simulink model "gm_external_state_machine"  (R2021a)
settings: Solver=FixedStepDiscrete  StartTime=0.0  StopTime=200*t_ADC  RelTol=1e-3
undefined symbols (not defined in the file or in its folder): A, IB, id_ref, iq_ref, ix_ref, iy_ref, lambda_d, lambda_q, lambda_u, lambda_x, lambda_y, Ld_over_LB, Lq_over_LB, n_rpm, omega_m, omegaB, p, psi_pm_over_psiB, Rs_over_ZB, t_ADC, t_clock, Ts_times_ZB_over_Ld, Ts_times_ZB_over_Lq, Ts_times_ZB_over_Lx, Ts_times_ZB_over_Ly, v_dc, VB
libraries: nesl_utility x38, fl_lib x30, simulink x19, ee_lib x14, hdlsllib x4, spsAlphaBetaZerotodq0Lib x1
(part 1 of 4)
settings Model: Creator=micha  LastModifiedBy=micha
settings SolverCC: AlgebraicLoopSolver=TrustRegion
settings DataIOCC: LimitDataPoints=on  SaveOutput=off  SaveTime=off
settings OptimizationCC: BlockReduction=off  ConditionallyExecuteInputs=off  DefaultParameterBehavior=Inlined  LifeSpan=inf
settings DebuggingCC: AlgebraicLoopMsg=error  InheritedTsInSrcMsg=none  SingleTaskRateTransMsg=error  AllowSymbolicDim=off  StrictBusMsg=ErrorOnBusTreatedAsVector  SFUnexpectedBacktrackingDiag=warning  SFNoUnconditionalDefaultTransitionDiag=warning  SFExecutionAtInitializationDiag=none  SFMachineParentedDataDiag=warning  ArithmeticOperatorsInVariantConditions=warning
settings HardwareCC: ProdBitPerPointer=32  ProdBitPerSizeT=32  ProdBitPerPtrDiffT=32  ProdLargestAtomicFloat=None  ProdIntDivRoundTo=Undefined  ProdEndianess=Unspecified  ProdWordSize=32  ProdHWDeviceType=ASIC/FPGA->ASIC/FPGA  ProdEqTarget=off
settings SFSimCC: SimUseLocalCustomCode=off  CustomCodeUndefinedFunction=UseInterfaceOnly
settings RTWCC: RTWUseLocalCustomCode=off
settings CodeAppCC: StateflowObjectComments=on
settings GRTTargetCC: TargetLangStandard=C89/C90 (ANSI)
settings ConfigComp: CovScope=ReferencedModels  CovMetricSettings=dw  CovSaveCumulativeToWorkspaceVar=on  CovSaveSingleToWorkspaceVar=on  CovExternalEMLEnable=off  CovSFcnEnable=off

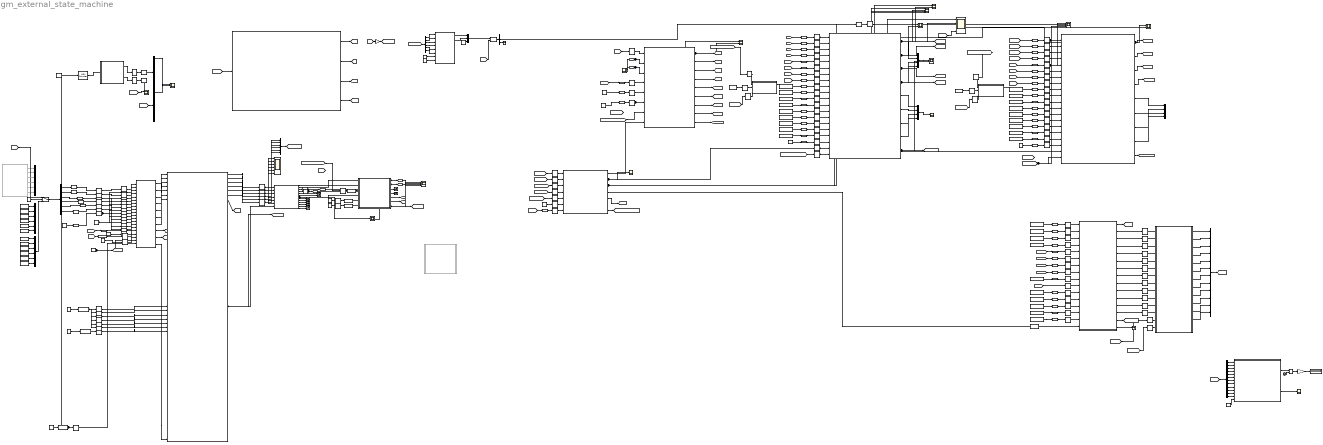
== system gm_external_state_machine ==
  note: 0=AXI 1=PL
  note: 1=sine source, 2=const
  note: check if timing is correct with delay done trigger
  note: 5 steps delay for xy currents, since dq transformation of alpha beta currents takes 5 clock steps. This way, the delay of dq is compensated
  6ph_PMSM_30deg_VSD1 : MATLAB Function  TreatAsAtomicUnit=on
  Alpha-Beta-Zero to dq1 : spsAlphaBetaZerotodq0Lib/Alpha-Beta-Zero to dq0  Alignment=Aligned with phase A axis
      settings: SourceProductBaseCode=PS
  Clock : Clock
  Constant : Constant  Value=64  OutDataTypeStr=uint32  SampleTime=-1
  Constant1 : Constant  Value=5
  Constant10 : Constant  Value=psi_pm_over_psiB
  Constant11 : Constant  Value=0.36
  Constant{12,45..50,52} (8 alike) : Constant  Value=0
  Constant13 : Constant  Value=5
  Constant14 : Constant  Value=psi_pm_over_psiB
  Constant15 : Constant  Value=Rs_over_ZB
  Constant16 : Constant  Value=omega_m/omegaB
  Constant17 : Constant  Value=Ts_times_ZB_over_Ld
  Constant18 : Constant  Value=Ts_times_ZB_over_Lq
  Constant19 : Constant  Value=Ts_times_ZB_over_Lx
  Constant{2,25,41,51} (4 alike) : Constant
  Constant20 : Constant  Value=Ts_times_ZB_over_Ly
  Constant21 : Constant  Value=Ld_over_LB
  Constant22 : Constant  Value=Lq_over_LB
  Constant23 : Constant  Value=omega_m/omegaB
  Constant24 : Constant  Value=1/3
  Constant26 : Constant  Value=v_dc
  Constant27 : Constant  Value=iq_ref/IB
  Constant28 : Constant  Value=ix_ref/IB
  Constant29 : Constant  Value=iy_ref/IB
  Constant3 : Constant  Value=Rs_over_ZB
  Constant30 : Constant  Value=0  SampleTime=-1
  Constant31 : Constant  Value=lambda_d
  Constant32 : Constant  Value=lambda_q
  Constant33 : Constant  Value=lambda_x
  Constant34 : Constant  Value=lambda_y
  Constant35 : Constant  Value=lambda_u
  Constant36 : Constant  Value=0.00785
  Constant37 : Constant  Value=-0.87
  Constant38 : Constant  Value=0.862
  Constant39 : Constant  Value=-0.493
  Constant4 : Constant  Value=Ts_times_ZB_over_Ld
  Constant40 : Constant  Value=-0.507
  Constant42 : Constant  Value=id_ref/IB
  Constant43 : Constant  SampleTime=-1
  Constant44 : Constant  Value=0.0  SampleTime=-1
  Constant5 : Constant  Value=Ts_times_ZB_over_Lq
  Constant53 : Constant  Value=1/omegaB  OutDataTypeStr=fixdt(0,18,18)
  Constant54 : Constant  Value=1/omegaB  OutDataTypeStr=fixdt(0,18,18)
  Constant55 : Constant  Value=0  OutDataTypeStr=fixdt(1,24,11)  SampleTime=-1
  Constant56 : Constant  Value=1/IB
  Constant57 : Constant  Value=1/VB
  Constant58 : Constant  Value=63
  Constant59 : Constant  OutDataTypeStr=boolean  SampleTime=-1
  Constant6 : Constant  Value=Ts_times_ZB_over_Lx
  Constant60 : Constant  Value=0  OutDataTypeStr=fixdt(1,27,15)  SampleTime=-1
  Constant61 : Constant  Value=0  OutDataTypeStr=fixdt(1,27,20)  SampleTime=-1
  Constant7 : Constant  Value=Ts_times_ZB_over_Ly
  Constant8 : Constant  Value=Ld_over_LB
  Constant9 : Constant  Value=Lq_over_LB
  Data Type Conversion{,3,55..58} (6 alike) : DataTypeConversion  OutDataTypeStr=fixdt_type_xy_currents
  Data Type Conversion1 : DataTypeConversion  OutDataTypeStr=boolean
  Data Type Conversion{2,6,10..11,13,65} (6 alike) : DataTypeConversion  OutDataTypeStr=fixdt_type_polepairs
  Data Type Conversion{12,14..28} (16 alike) : DataTypeConversion  OutDataTypeStr=fixdt_type_constants
  Data Type Conversion29 : DataTypeConversion  OutDataTypeStr=fixdt_type_speed
  Data Type Conversion30 : DataTypeConversion  OutDataTypeStr=fixdt_type_speed
  Data Type Conversion{4..5,31,43..45,50..53} (10 alike) : DataTypeConversion  OutDataTypeStr=fixdt_type_dq_currents
  Data Type Conversion32 : DataTypeConversion  OutDataTypeStr=fixdt(0,18,18)
  Data Type Conversion33 : DataTypeConversion  OutDataTypeStr=fixdt(0,18,18)
  Data Type Conversion{34..36,38,40,67..68} (7 alike) : DataTypeConversion  OutDataTypeStr=fixdt(1,27,15)
  Data Type Conversion37 : DataTypeConversion  OutDataTypeStr=fixdt(1,27,20)
  Data Type Conversion39 : DataTypeConversion  OutDataTypeStr=fixdt(1,18,14)
  Data Type Conversion{7..8,41..42,46..49} (8 alike) : DataTypeConversion  OutDataTypeStr=fixdt_type_dqxy_voltages
  Data Type Conversion54 : DataTypeConversion  OutDataTypeStr=fixdt_type_max_current
  Data Type Conversion59 : DataTypeConversion  OutDataTypeStr=fixdt(1,18,14)
  Data Type Conversion{60..64} (5 alike) : DataTypeConversion  OutDataTypeStr=fixdt_type_lambda
  Data Type Conversion69 : DataTypeConversion  OutDataTypeStr=fixdt(1,24,11)
  Data Type Conversion9 : DataTypeConversion  OutDataTypeStr=fixdt(1,27,20)
  Delay : Delay  DelayLength=10
  Delay1 : Delay  DelayLength=46
  Delay2 : Delay  DelayLength=46
  Delay3 : Delay  DelayLength=5
  Delay4 : Delay  DelayLength=5
  Delay5 : Delay  DelayLength=1
  Demux : Demux  Outputs=6
  Demux1 : Demux  Outputs=12
  Demux2 : Demux  Outputs=12
  Demux3 : Demux  Outputs=12
  Demux4 : Demux  Outputs=3
  Demux5 : Demux  Outputs=6
  Display : Display
  Divide : Product  Inputs=*/
  Gain : Gain  Gain=1/IB
  Gain19 : Gain  Gain=1/(12*2)
  HDL Counter : hdlsllib/Sources/HDL Counter  CountType=Count limited  CountInit=1  CountStep=1  CountMax=100  CountFromType=Initial value  CountFrom=1  CountResetPort=off  CountLoadPort=off  CountEnbPort=on  CountDirPort=off  CountHitOutputPort=off  CountDataType=Unsigned  CountWordLen=8  CountFracLen=0  CountSampTime=1
  MATLAB Function : MATLAB Function  TreatAsAtomicUnit=on
  Mux : Mux
  Mux1 : Mux
  Mux2 : Mux  Inputs=12
  Mux3 : Mux
  Mux{4,6..7,9} (4 alike) : Mux  Inputs=6
  Mux5 : Mux  Inputs=3
  Pulse Generator2 : DiscretePulseGenerator  PulseType=Time based  Period=t_ADC  PulseWidth=5
  Rate Transition{,1..10,12..54,56..67,69..74,77..128} (124 alike) : RateTransition  OutPortSampleTime=t_clock
  Rate Transition{11,55,68,75..76} (5 alike) : RateTransition  InitialCondition=1  OutPortSampleTime=t_clock
  Scope : Scope  NumInputPorts=5
  Scope1 : Scope  NumInputPorts=4
  Scope{3..5,9..12} (7 alike) : Scope  NumInputPorts=2
  Scope13 : Scope
  Scope2 : Scope  NumInputPorts=3
  Scope6 : Scope  NumInputPorts=4
  Scope7 : Scope  NumInputPorts=4
  Scope8 : Scope
  Subsystem : Subsystem  Commented=on
  Subsystem1 : Subsystem
  Subsystem2 : Subsystem
  Switch : Switch  Criteria=u2 > Threshold
  Terminator{,1..11} (12 alike) : Terminator
  cost_opt : Subsystem  TreatAsAtomicUnit=on
  ctrl_state_machine : Subsystem  TreatAsAtomicUnit=on
  delay_comp : Subsystem  TreatAsAtomicUnit=on
  i_delay : Scope  NumInputPorts=2
  mpc_enable : Subsystem
  natural values : Scope  NumInputPorts=6
  prediction : Subsystem  TreatAsAtomicUnit=on
  pu_omega_m : Subsystem  TreatAsAtomicUnit=on
  pu_omega_m1 : Subsystem
  pu_voltages_vsd : Subsystem  TreatAsAtomicUnit=on
  switchNumb : Scope
  uz_debug_switch_measurements : Subsystem  TreatAsAtomicUnit=on
  uz_park_transformation : Subsystem  TreatAsAtomicUnit=on
  uz_park_transformation_old : Subsystem  Commented=on  TreatAsAtomicUnit=on
  uz_pu_conversion : Subsystem  TreatAsAtomicUnit=on
  uz_vsd_6ph_30deg : Subsystem  TreatAsAtomicUnit=on
  wires:
  uz_debug_switch_measurements/9(out8) -> [theta_el_from_debug_switch]
  Rate Transition128/1 -> uz_debug_switch_measurements/18(in0_AXI8)
  Constant61/1 -> Rate Transition128/1
  Rate Transition127/1 -> uz_debug_switch_measurements/17(in8)
  Data Type Conversion37/1 -> Rate Transition127/1
  [theta_el] -> Data Type Conversion37/1
  Constant55/1 -> Rate Transition126/1
  Data Type Conversion69/1 -> Rate Transition125/1
  uz_debug_switch_measurements/8(out7) -> [omega_m_from_debug_switch]
  [omega_m] -> Data Type Conversion69/1
  Rate Transition126/1 -> uz_debug_switch_measurements/16(in0_AXI7)
  Rate Transition125/1 -> uz_debug_switch_measurements/15(in7)
  Constant60/1 -> Rate Transition120/1, Rate Transition118/1, Rate Transition116/1, Rate Transition111/1, Rate Transition113/1, Rate Transition122/1
  Rate Transition124/1 -> uz_debug_switch_measurements/14(in0_AXI6)
  Rate Transition123/1 -> uz_debug_switch_measurements/13(in6)
  Rate Transition122/1 -> uz_debug_switch_measurements/12(in0_AXI5)
  Rate Transition121/1 -> uz_debug_switch_measurements/11(in5)
  Rate Transition120/1 -> uz_debug_switch_measurements/10(in0_AXI4)
  Rate Transition119/1 -> uz_debug_switch_measurements/9(in4)
  Rate Transition118/1 -> uz_debug_switch_measurements/8(in0_AXI3)
  Rate Transition117/1 -> uz_debug_switch_measurements/7(in3)
  Rate Transition116/1 -> uz_debug_switch_measurements/6(in0_AXI2)
  Rate Transition115/1 -> uz_debug_switch_measurements/3(in1)
  Rate Transition114/1 -> uz_debug_switch_measurements/5(in2)
  Rate Transition113/1 -> uz_debug_switch_measurements/4(in0_AXI1)
  Rate Transition112/1 -> uz_debug_switch_measurements/1(in0)
  Rate Transition111/1 -> uz_debug_switch_measurements/2(in0_AXI)
  Constant59/1 -> uz_debug_switch_measurements/19(real_or_debug_AXI), [debug_enb]
  uz_debug_switch_measurements/10(debug_ip_done) -> uz_pu_conversion/65(adc_valid_trigger)
  Rate Transition10/1 -> uz_debug_switch_measurements/20(adc_valid_trigger)
  uz_debug_switch_measurements/7(out6) -> uz_pu_conversion/7(in6)
  Rate Transition103/1 -> Rate Transition123/1, Rate Transition124/1
  Rate Transition97/1 -> Rate Transition121/1
  Rate Transition98/1 -> Rate Transition119/1
  Rate Transition99/1 -> Rate Transition117/1
  Rate Transition100/1 -> Rate Transition114/1
  Rate Transition101/1 -> Rate Transition115/1
  Rate Transition102/1 -> Rate Transition112/1
  uz_debug_switch_measurements/6(out5) -> uz_pu_conversion/6(in5)
  uz_debug_switch_measurements/5(out4) -> uz_pu_conversion/5(in4)
  uz_debug_switch_measurements/4(out3) -> uz_pu_conversion/4(in3)
  uz_debug_switch_measurements/3(out2) -> uz_pu_conversion/3(in2)
  uz_debug_switch_measurements/2(out1) -> uz_pu_conversion/2(in1)
  uz_debug_switch_measurements/1(out0) -> uz_pu_conversion/1(in0)
  uz_pu_conversion/6(out5) -> Rate Transition37/1
  uz_pu_conversion/5(out4) -> Rate Transition36/1
  uz_pu_conversion/4(out3) -> Rate Transition34/1
  uz_pu_conversion/3(out2) -> Rate Transition33/1
  uz_pu_conversion/2(out1) -> Rate Transition32/1
  uz_pu_conversion/1(out0) -> Rate Transition35/1
  Mux1/1 -> Scope13/1
  Constant58/1 -> Data Type Conversion65/1
  uz_pu_conversion/7(out6) -> [v_dc_pu]
  Data Type Conversion68/1 -> Rate Transition103/1
  Data Type Conversion67/1 -> Rate Transition97/1
  Data Type Conversion40/1 -> Rate Transition98/1
  Data Type Conversion38/1 -> Rate Transition99/1
  Data Type Conversion36/1 -> Rate Transition100/1
  Data Type Conversion35/1 -> Rate Transition101/1
  Data Type Conversion34/1 -> Rate Transition102/1
  Data Type Conversion33/1 -> Rate Transition106/1, Rate Transition108/1, Rate Transition109/1, Rate Transition110/1, Rate Transition104/1, Rate Transition105/1
  Data Type Conversion32/1 -> Rate Transition107/1
  Constant57/1 -> Data Type Conversion32/1
  Constant56/1 -> Data Type Conversion33/1
  Rate Transition107/1 -> uz_pu_conversion/39(AXI_pu_conv_in6)
  Rate Transition108/1 -> uz_pu_conversion/38(AXI_pu_conv_in5)
  Rate Transition109/1 -> uz_pu_conversion/37(AXI_pu_conv_in4)
  Rate Transition110/1 -> uz_pu_conversion/36(AXI_pu_conv_in3)
  Rate Transition104/1 -> uz_pu_conversion/35(AXI_pu_conv_in2)
  Rate Transition105/1 -> uz_pu_conversion/34(AXI_pu_conv_in1)
  Rate Transition106/1 -> uz_pu_conversion/33(AXI_pu_conv_in0)
  Constant26/1 -> Data Type Conversion68/1
  Rate Transition96/1 -> mpc_enable/2(G1)
  Rate Transition95/1 -> mpc_enable/1(G0)
  Rate Transition93/1 -> mpc_enable/3(G2)
  Rate Transition94/1 -> mpc_enable/4(G3)
  Rate Transition92/1 -> mpc_enable/6(G5)
  Rate Transition91/1 -> mpc_enable/5(G4)
  Rate Transition90/1 -> mpc_enable/8(G7)
  Rate Transition89/1 -> mpc_enable/7(G6)
  Rate Transition88/1 -> mpc_enable/10(G9)
  Rate Transition87/1 -> mpc_enable/9(G8)
  Rate Transition86/1 -> mpc_enable/14(adc_valid_trigger)
  Rate Transition85/1 -> mpc_enable/13(AXI_mpc_enb)
  Rate Transition84/1 -> mpc_enable/12(G11)
  Rate Transition83/1 -> mpc_enable/11(G10)
  [debug_enb] -> Rate Transition85/1
  [pu_conv_valid] -> Rate Transition86/1
  cost_opt/2(G0) -> Rate Transition95/1
  cost_opt/3(G1) -> Rate Transition96/1
  cost_opt/4(G2) -> Rate Transition93/1
  cost_opt/5(G3) -> Rate Transition94/1
  cost_opt/6(G4) -> Rate Transition91/1
  cost_opt/7(G5) -> Rate Transition92/1
  cost_opt/8(G6) -> Rate Transition89/1
  cost_opt/9(G7) -> Rate Transition90/1
  cost_opt/10(G8) -> Rate Transition87/1
  cost_opt/11(G9) -> Rate Transition88/1
  cost_opt/12(G10) -> Rate Transition83/1
  cost_opt/13(G11) -> Rate Transition84/1
  mpc_enable/8(out_G7) -> Mux2/8
  mpc_enable/4(out_G3) -> Mux2/4
  mpc_enable/9(out_G8) -> Mux2/9
  mpc_enable/11(out_G10) -> Mux2/11
  mpc_enable/7(out_G6) -> Mux2/7
  mpc_enable/12(out_G11) -> Mux2/12
  mpc_enable/6(out_G5) -> Mux2/6
  mpc_enable/3(out_G2) -> Mux2/3
  mpc_enable/5(out_G4) -> Mux2/5
  mpc_enable/2(out_G1) -> Mux2/2
  mpc_enable/1(out_G0) -> Mux2/1
  Mux2/1 -> [opt_gates]
  mpc_enable/10(out_G9) -> Mux2/10
  [omega_m_from_debug_switch] -> Rate Transition82/1
  Rate Transition81/1 -> pu_omega_m1/2(AXI_pu_conv_in)
  Constant54/1 -> Rate Transition81/1
  [pu_conv_valid] -> Rate Transition80/1
  Rate Transition82/1 -> pu_omega_m1/1(in1)
  Rate Transition80/1 -> pu_omega_m1/3(adc_valid_trigger)
  Rate Transition79/1 -> pu_omega_m/1(in1)
  Rate Transition78/1 -> pu_omega_m/2(AXI_pu_conv_in)
  Rate Transition77/1 -> pu_omega_m/3(adc_valid_trigger)
  Constant53/1 -> Rate Transition78/1
  [pu_conv_valid] -> Rate Transition77/1
  [omega_m_from_debug_switch] -> Rate Transition79/1
  Delay5/1 -> Rate Transition8/1
  Rate Transition8/1 -> Scope9/1
  Demux4/2 -> Delay5/1  "id"
  Demux4/3 -> Terminator11/1
  6ph_PMSM_30deg_VSD1/2(y2) -> Mux5/2  "beta"
  Alpha-Beta-Zero to dq1/1 -> Demux4/1
  Mux5/1 -> Alpha-Beta-Zero to dq1/1
  6ph_PMSM_30deg_VSD1/1(y1) -> Mux5/1  "alpha"
  [theta_el] -> Alpha-Beta-Zero to dq1/2
  Constant52/1 -> Mux5/3
  Gain/1 -> [pu_phase_currents]
  [i_ph] -> Gain/1
  Demux5/6 -> 6ph_PMSM_30deg_VSD1/6(u6)
  Demux5/1 -> 6ph_PMSM_30deg_VSD1/1(u1)
  Constant24/1 -> 6ph_PMSM_30deg_VSD1/7(k6)
  [pu_phase_currents] -> Demux5/1
  Constant51/1 -> 6ph_PMSM_30deg_VSD1/8(c6)
  Demux5/3 -> 6ph_PMSM_30deg_VSD1/3(u3)
  Demux5/2 -> 6ph_PMSM_30deg_VSD1/2(u2)
  Demux5/5 -> 6ph_PMSM_30deg_VSD1/5(u5)
  Demux5/4 -> 6ph_PMSM_30deg_VSD1/4(u4)
  Delay4/1 -> Scope/4, [iy_pu]
  Delay3/1 -> [ix_pu], Scope/3
  Mux/1 -> i_delay/1
  Rate Transition7/1 -> delay_comp/19(trigger_delay_comp), Scope7/4
  Rate Transition6/1 -> delay_comp/20(trigger_park_done), Scope7/3
  [trigger_park_done_statemachine] -> Rate Transition6/1
  ctrl_state_machine/7(trigger_park_done_statemachine) -> [trigger_park_done_statemachine]
  delay_comp/3(ix_delay_pu) -> Mux/3, [ix_delay_pu]
  delay_comp/4(iy_delay_pu) -> Mux/4, [iy_delay_pu]
  delay_comp/2(iq_delay_pu) -> Mux/2, [iq_delay_pu], Scope9/2
  delay_comp/1(id_delay_pu) -> Mux/1, [id_delay_pu], Scope1/2, Scope7/2, Scope11/2  "id_delay"
  [opt_gates] -> Subsystem1/1(In1)
  Delay2/1 -> Scope3/2
  [opt_index] -> Scope3/1
  MATLAB Function/2(opt_idx) -> Rate Transition5/1
  Rate Transition5/1 -> Delay2/1
  Rate Transition/1 -> Delay1/1
  MATLAB Function/1(G_opt) -> Rate Transition/1
  Demux3/1 -> Scope2/1
  Demux1/1 -> Scope2/2
  [opt_gates] -> Demux3/1
  Delay/1 -> HDL Counter/1
  HDL Counter/1 -> MATLAB Function/1(u)
  Delay1/1 -> Demux1/1
  [opt_index] -> Scope1/4
  Rate Transition41/1 -> delay_comp/1(id_pu), Scope1/1, Scope7/1, Scope10/2, Scope11/1  "id_measured"
  Mux4/1 -> [meas_pu_currents]
  Rate Transition37/1 -> natural values/6, Mux4/6, uz_vsd_6ph_30deg/6(c2)
  ctrl_state_machine/5(index) -> [index]
  [trigger_park_done_statemachine] -> pu_voltages_vsd/7(trigger_park_done)
  [delay_comp_done] -> prediction/20(trigger_delay_comp_done), Scope6/4
  ctrl_state_machine/3(trigger_prediction) -> prediction/19(trigger_prediction), Scope6/2
  ctrl_state_machine/2(trigger_delay_comp) -> Rate Transition7/1, Scope8/1
  ctrl_state_machine/1(trigger_voltages) -> pu_voltages_vsd/8(trigger_voltages)
  [trigger_park_done] -> Rate Transition58/1
  Constant29/1 -> Data Type Conversion56/1
  Rate Transition39/1 -> delay_comp/11(Ts_times_ZB_over_Ld_AXI)
  prediction/5(id_pred_pu_AXI) -> Mux3/1
  Rate Transition62/1 -> cost_opt/9(max_current_pu_AXI)
  Data Type Conversion29/1 -> Rate Transition43/1
  Rate Transition49/1 -> prediction/3(ix_delay_pu)
  Rate Transition45/1 -> delay_comp/2(iq_pu)
  pu_omega_m/1(out1) -> Data Type Conversion29/1
  Constant7/1 -> Data Type Conversion24/1
  Data Type Conversion7/1 -> Rate Transition67/1
  Data Type Conversion50/1 -> Rate Transition59/1
  Demux2/9 -> Subsystem2/9(ss_in_8)
  Rate Transition56/1 -> cost_opt/8(iy_pred_pu)
  Data Type Conversion25/1 -> Rate Transition29/1
  delay_comp/8(iy_delay_pu_AXI) -> Mux1/4
  Rate Transition30/1 -> delay_comp/16(Lq_over_LB_AXI)
  Constant31/1 -> Data Type Conversion60/1
  Rate Transition14/1 -> prediction/13(Ts_times_ZB_over_Lx_AXI)
  Rate Transition42/1 -> delay_comp/12(Ts_times_ZB_over_Lq_AXI)
  Rate Transition27/1 -> delay_comp/14(Ts_times_ZB_over_Ly_AXI)
  Data Type Conversion26/1 -> Rate Transition30/1
  Constant3/1 -> Data Type Conversion20/1
  Data Type Conversion23/1 -> Rate Transition26/1
  Data Type Conversion5/1 -> Rate Transition45/1
  [vy_pu] -> Data Type Conversion47/1
  Demux2/5 -> Subsystem2/5(ss_in_4)
  Rate Transition25/1 -> delay_comp/10(Rs_over_ZB_AXI)
  Data Type Conversion/1 -> Rate Transition44/1
  Constant28/1 -> Data Type Conversion55/1
  prediction/1(id_pred_pu) -> [id_pred_pu], Scope1/3, Scope10/1
  Data Type Conversion2/1 -> Rate Transition11/1
  [vq_pu] -> Data Type Conversion49/1
  [iy_pred_pu] -> Data Type Conversion51/1
  [vx_pu] -> Data Type Conversion46/1
  Data Type Conversion24/1 -> Rate Transition27/1
  prediction/3(ix_pred_pu) -> [ix_pred_pu]
  Data Type Conversion54/1 -> Rate Transition62/1
  [ix_pu] -> Data Type Conversion/1
  Subsystem2/2(switchNumb) -> switchNumb/1
  Data Type Conversion53/1 -> Rate Transition60/1
  [ix_delay_pu] -> Data Type Conversion31/1
  Rate Transition66/1 -> cost_opt/2(iq_ref_pu_AXI)
  [iy_delay_pu] -> Data Type Conversion43/1
  Data Type Conversion62/1 -> Rate Transition71/1
  [id_pu] -> Data Type Conversion4/1
  [id_delay_pu] -> Data Type Conversion44/1
  Data Type Conversion8/1 -> Rate Transition74/1
  Data Type Conversion49/1 -> Rate Transition54/1
  Data Type Conversion52/1 -> Rate Transition57/1
  Rate Transition31/1 -> delay_comp/17(psi_pm_over_psiB_AXI)
  [id_pred_pu] -> Data Type Conversion52/1
  [ix_pred_pu] -> Data Type Conversion50/1
  Data Type Conversion44/1 -> Rate Transition28/1
  Data Type Conversion55/1 -> Rate Transition63/1
  Rate Transition59/1 -> cost_opt/7(ix_pred_pu)
  Constant6/1 -> Data Type Conversion23/1
  Data Type Conversion63/1 -> Rate Transition72/1
  Rate Transition55/1 -> Scope4/1, pu_voltages_vsd/6(index_AXI)
  Rate Transition28/1 -> prediction/1(id_delay_pu), Scope6/3
  [iq_pred_pu] -> Data Type Conversion53/1
  Data Type Conversion6/1 -> Rate Transition75/1
  Constant27/1 -> Data Type Conversion58/1
  Rate Transition23/1 -> prediction/9(omega_m_pu)
  Rate Transition57/1 -> cost_opt/5(id_pred_pu)
  [vx_pu] -> Data Type Conversion41/1
  Divide/1 -> Gain19/1
  [vy_pu] -> Data Type Conversion42/1
  Rate Transition16/1 -> prediction/14(Ts_times_ZB_over_Ly_AXI)
  Rate Transition65/1 -> cost_opt/1(id_ref_pu_AXI)
  Rate Transition64/1 -> cost_opt/4(iy_ref_pu_AXI)
  Constant5/1 -> Data Type Conversion22/1
  Rate Transition63/1 -> cost_opt/3(ix_ref_pu_AXI)
  Rate Transition72/1 -> cost_opt/14(lambda_y_AXI)
  Rate Transition71/1 -> cost_opt/13(lambda_x_AXI)
  Constant42/1 -> Data Type Conversion57/1
  Data Type Conversion60/1 -> Rate Transition69/1
  Rate Transition76/1 -> ctrl_state_machine/7(last_opt_index)
  Data Type Conversion22/1 -> Rate Transition42/1
  Data Type Conversion61/1 -> Rate Transition70/1
  Demux2/4 -> Subsystem2/4(ss_in_3)
  Data Type Conversion64/1 -> Rate Transition73/1
  Rate Transition73/1 -> cost_opt/15(lambda_u_AXI)
  Constant4/1 -> Data Type Conversion21/1
  Constant35/1 -> Data Type Conversion64/1
  Data Type Conversion56/1 -> Rate Transition64/1
  cost_opt/14(optimization_done) -> [optimization_done]  "optimization done"
  Rate Transition60/1 -> cost_opt/6(iq_pred_pu)
  Data Type Conversion20/1 -> Rate Transition25/1
  Constant34/1 -> Data Type Conversion63/1
  [iq_pu] -> Data Type Conversion5/1
  Rate Transition13/1 -> prediction/10(Rs_over_ZB_AXI)
  cost_opt/1(opt_index) -> [opt_index]  "result"
  Rate Transition53/1 -> prediction/5(vd_pu), Scope6/1
  Constant33/1 -> Data Type Conversion62/1
  prediction/9(prediction_done) -> [prediction_done]
  Constant1/1 -> Data Type Conversion13/1
  Data Type Conversion3/1 -> Rate Transition22/1
  Data Type Conversion46/1 -> Rate Transition51/1
  Data Type Conversion17/1 -> Rate Transition16/1
  [vd_pu] -> Data Type Conversion48/1
  [iy_pu] -> Data Type Conversion3/1
  Data Type Conversion51/1 -> Rate Transition56/1
  Constant10/1 -> Data Type Conversion28/1
  Data Type Conversion11/1 -> Rate Transition12/1
  Rate Transition43/1 -> delay_comp/9(omega_m_pu)
  Rate Transition22/1 -> delay_comp/4(iy_pu)
  [opt_index] -> Data Type Conversion10/1
  Data Type Conversion13/1 -> Rate Transition15/1
  pu_voltages_vsd/4(pu_vy) -> [vy_pu]
  Rate Transition17/1 -> prediction/15(Ld_over_LB_AXI)
  Rate Transition29/1 -> delay_comp/15(Ld_over_LB_AXI)
  Rate Transition20/1 -> prediction/11(Ts_times_ZB_over_Ld_AXI)
  Rate Transition12/1 -> prediction/18(polepairs_AXI)
  Data Type Conversion48/1 -> Rate Transition53/1
  Constant19/1 -> Data Type Conversion16/1
  Data Type Conversion10/1 -> Rate Transition76/1
  Data Type Conversion19/1 -> Rate Transition18/1
  Constant11/1 -> Data Type Conversion54/1
  Constant32/1 -> Data Type Conversion61/1
  Data Type Conversion43/1 -> Rate Transition24/1
  [vd_pu] -> Data Type Conversion7/1
  pu_voltages_vsd/8(pu_vy_AXI) -> [vy_pu_AXI]
  Data Type Conversion27/1 -> Rate Transition19/1
  [index] -> Rate Transition68/1
  pu_voltages_vsd/6(pu_vq_AXI) -> [vq_pu_AXI]
  ctrl_state_machine/4(trigger_optimization) -> cost_opt/16(trigger_optimization)
  Rate Transition70/1 -> cost_opt/12(lambda_q_AXI)
  pu_voltages_vsd/7(pu_vx_AXI) -> [vx_pu_AXI]
  Demux2/8 -> Subsystem2/8(ss_in_7)
  prediction/4(iy_pred_pu) -> [iy_pred_pu]
  Demux2/7 -> Subsystem2/7(ss_in_6)
  [sin] -> pu_voltages_vsd/2(sin_angle), Scope5/1
  Rate Transition54/1 -> prediction/6(vq_pu)
  Rate Transition69/1 -> cost_opt/11(lambda_d_AXI)
  Demux2/12 -> Subsystem2/12(ss_in_11)
  Data Type Conversion28/1 -> Rate Transition31/1
  Gain19/1 -> Display/1
  prediction/6(iq_pred_pu_AXI) -> Mux3/2
  Constant20/1 -> Data Type Conversion17/1
  Demux2/6 -> Subsystem2/6(ss_in_5)
  Rate Transition11/1 -> pu_voltages_vsd/5(index_select_AXI)
  Data Type Conversion57/1 -> Rate Transition65/1
  pu_voltages_vsd/3(pu_vx) -> [vx_pu]
  Rate Transition52/1 -> prediction/8(vy_pu)
  Rate Transition68/1 -> cost_opt/10(index)
  Rate Transition18/1 -> prediction/16(Lq_over_LB_AXI)
  Demux2/1 -> Subsystem2/1(ss_in_0)
  [index] -> Data Type Conversion6/1
  Data Type Conversion4/1 -> Rate Transition41/1
  prediction/2(iq_pred_pu) -> [iq_pred_pu]
  Data Type Conversion58/1 -> Rate Transition66/1
  Demux2/10 -> Subsystem2/10(ss_in_9)
  Demux2/3 -> Subsystem2/3(ss_in_2)
  Data Type Conversion42/1 -> Rate Transition48/1
  prediction/8(iy_pred_pu_AXI) -> Mux3/4
  Clock/1 -> Divide/2
  Constant9/1 -> Data Type Conversion26/1
  Rate Transition44/1 -> delay_comp/3(ix_pu)
  Demux2/2 -> Subsystem2/2(ss_in_1)
  Data Type Conversion30/1 -> Rate Transition23/1
  prediction/7(ix_pred_pu_AXI) -> Mux3/3
  [opt_gates] -> Demux2/1
  Demux2/11 -> Subsystem2/11(ss_in_10)
  Rate Transition67/1 -> delay_comp/5(vd_pu)
  cost_opt/15(costs) -> Terminator10/1
  Rate Transition50/1 -> prediction/2(iq_delay_pu)
  Data Type Conversion47/1 -> Rate Transition52/1
  pu_voltages_vsd/5(pu_vd_AXI) -> [vd_pu_AXI]
  Constant17/1 -> Data Type Conversion14/1
  Rate Transition21/1 -> prediction/12(Ts_times_ZB_over_Lq_AXI)
  Rate Transition48/1 -> delay_comp/8(vy_pu)
  Subsystem2/1(switchNumb_AXI) -> Divide/1
  Data Type Conversion15/1 -> Rate Transition21/1
  [iq_delay_pu] -> Data Type Conversion45/1
  Data Type Conversion31/1 -> Rate Transition49/1
  Constant30/1 -> Subsystem2/13(bResetAXI)
  Rate Transition46/1 -> pu_voltages_vsd/1(v_DC_pu)
  [cos] -> pu_voltages_vsd/3(cos_angle), Scope5/2
  Constant2/1 -> Data Type Conversion2/1
  Rate Transition26/1 -> delay_comp/13(Ts_times_ZB_over_Lx_AXI)
  Rate Transition24/1 -> prediction/4(iy_delay_pu)
  Data Type Conversion45/1 -> Rate Transition50/1
  pu_voltages_vsd/2(pu_vq) -> [vq_pu]
  Data Type Conversion18/1 -> Rate Transition17/1
  delay_comp/9(delay_comp_done) -> [delay_comp_done], i_delay/2
  [vq_pu] -> Data Type Conversion8/1
  delay_comp/5(id_delay_pu_AXI) -> Mux1/1
  Rate Transition75/1 -> pu_voltages_vsd/4(index)
  Constant8/1 -> Data Type Conversion25/1
  Data Type Conversion21/1 -> Rate Transition39/1
  pu_omega_m1/1(out1) -> Data Type Conversion30/1
  Constant18/1 -> Data Type Conversion15/1
  Constant21/1 -> Data Type Conversion18/1
  Constant15/1 -> Data Type Conversion12/1
  Rate Transition19/1 -> prediction/17(psi_pm_over_psiB_AXI)
  Data Type Conversion14/1 -> Rate Transition20/1
  delay_comp/6(iq_delay_pu_AXI) -> Mux1/2
  Rate Transition51/1 -> prediction/7(vx_pu)
  Data Type Conversion41/1 -> Rate Transition47/1
  Rate Transition47/1 -> delay_comp/7(vx_pu)
  Rate Transition74/1 -> delay_comp/6(vq_pu)
  Constant22/1 -> Data Type Conversion19/1
  [v_dc_pu] -> Rate Transition46/1
  pu_voltages_vsd/1(pu_vd) -> [vd_pu], Scope4/2
  pu_voltages_vsd/9(voltages_done) -> [voltages_done]  "calc_done"
  Rate Transition15/1 -> delay_comp/18(polepairs_AXI)
  Data Type Conversion65/1 -> Rate Transition55/1
  delay_comp/7(ix_delay_pu_AXI) -> Mux1/3
  Data Type Conversion12/1 -> Rate Transition13/1
  Data Type Conversion16/1 -> Rate Transition14/1
  Constant14/1 -> Data Type Conversion27/1
  Constant13/1 -> Data Type Conversion11/1
  uz_park_transformation/4(y2_AXI) -> Terminator9/1
  Subsystem/2(output1) -> Mux6/2
  [theta_el_from_debug_switch] -> Rate Transition38/1
  uz_park_transformation/6(cos) -> [cos]
  Pulse Generator2/1 -> Data Type Conversion1/1
  Constant49/1 -> Mux9/5
  Rate Transition34/1 -> uz_vsd_6ph_30deg/4(a2), natural values/4, Mux4/4
  Constant40/1 -> Mux7/5
  uz_vsd_6ph_30deg/11(y_AXI) -> Terminator5/1
  Data Type Conversion1/1 -> Rate Transition10/1, Delay/1
  uz_pu_conversion/33(pu_conv_done) -> uz_vsd_6ph_30deg/7(pu_conv_valid), [pu_conv_valid]
  Demux/1 -> Data Type Conversion34/1
  Rate Transition32/1 -> uz_vsd_6ph_30deg/2(b1), natural values/2, Mux4/2
  Constant41/1 -> Mux7/6
  Demux/3 -> Data Type Conversion36/1
  Subsystem/5(output4) -> Mux6/5
  Demux/5 -> Data Type Conversion40/1
  Demux/6 -> Data Type Conversion67/1
  Constant25/1 -> Rate Transition40/1
  Subsystem/6(output5) -> Mux6/6
  Constant50/1 -> Mux9/6
  Constant39/1 -> Mux7/4
  Constant43/1 -> Switch/2
  Rate Transition35/1 -> uz_vsd_6ph_30deg/1(a1), natural values/1, Mux4/1
  Switch/1 -> Demux/1
  Constant36/1 -> Mux7/1
  Constant37/1 -> Mux7/2
  Constant47/1 -> Mux9/3
  uz_vsd_6ph_30deg/12(z1_AXI) -> Terminator6/1
  Subsystem1/1(i_ph) -> [i_ph]
  uz_park_transformation/5(sin) -> [sin]
  Constant45/1 -> Mux9/1
  Subsystem/1(output) -> Mux6/1
  uz_vsd_6ph_30deg/9(beta_AXI) -> Terminator3/1
  Constant48/1 -> Mux9/4
  Subsystem1/2(i_dc) -> [i_dc]
  Subsystem1/3(theta_el) -> [theta_el]
  Mux9/1 -> Switch/3
  Subsystem1/4(omega_m) -> [omega_m]
  uz_vsd_6ph_30deg/10(x_AXI) -> Terminator4/1
  [i_ph] -> Switch/1
  Subsystem/3(output2) -> Mux6/3
  uz_park_transformation/1(y1) -> [id_pu], Scope/1  "id_pu"
  Rate Transition33/1 -> uz_vsd_6ph_30deg/3(c1), natural values/3, Mux4/3
  Demux/2 -> Data Type Conversion35/1
  uz_vsd_6ph_30deg/13(z2_AXI) -> Terminator7/1
  Constant38/1 -> Mux7/3
  uz_vsd_6ph_30deg/6(z2) -> Terminator1/1
  uz_vsd_6ph_30deg/5(z1) -> Terminator/1
  Subsystem/4(output3) -> Mux6/4
  Constant12/1 -> Rate Transition61/1
  uz_vsd_6ph_30deg/4(y1) -> Delay4/1
  Rate Transition40/1 -> Data Type Conversion39/1
  Rate Transition61/1 -> Data Type Conversion59/1
  Demux/4 -> Data Type Conversion38/1
  Constant46/1 -> Mux9/2
  uz_vsd_6ph_30deg/3(x1) -> Delay3/1
  Data Type Conversion59/1 -> uz_park_transformation/6(offset_angle_el_AXI)
  uz_park_transformation/2(y2) -> [iq_pu], Scope/2  "iq_pu"
  Data Type Conversion9/1 -> uz_park_transformation/3(angle_el)
  uz_vsd_6ph_30deg/8(alpha_AXI) -> Terminator2/1
  uz_park_transformation/3(y1_AXI) -> Terminator8/1
  uz_vsd_6ph_30deg/2(beta) -> uz_park_transformation/2(u2)
  uz_vsd_6ph_30deg/7(vsd_done) -> Scope12/1, uz_park_transformation/4(trigger)
  uz_vsd_6ph_30deg/1(alpha) -> uz_park_transformation/1(u1)
  Data Type Conversion39/1 -> uz_park_transformation/5(factor_angle_el_AXI)
  Rate Transition38/1 -> Data Type Conversion9/1
  Rate Transition36/1 -> uz_vsd_6ph_30deg/5(b2), natural values/5, Mux4/5
  uz_park_transformation/7(park_done) -> [trigger_park_done], Scope/5, Scope12/2  "calc_done"
  Constant/1 -> Rate Transition9/1
  Rate Transition9/1 -> ctrl_state_machine/6(AXI_no_of_iterations)  "opt_done"
  Rate Transition4/1 -> ctrl_state_machine/5(trigger_optimization_done)  "opt_done"
  Rate Transition3/1 -> ctrl_state_machine/4(trigger_prediction_done)  "pred_done"
  Rate Transition2/1 -> ctrl_state_machine/3(trigger_delay_comp_done)  "delay_done"
  Rate Transition1/1 -> ctrl_state_machine/2(trigger_voltages_done)  "volts_done"
  Rate Transition58/1 -> ctrl_state_machine/1(trigger_start_state_machine)  "park_done"
  [voltages_done] -> Rate Transition1/1
  [delay_comp_done] -> Rate Transition2/1
  [prediction_done] -> Rate Transition3/1
  [optimization_done] -> Rate Transition4/1

== system gm_external_state_machine/Subsystem ==
  Electrical Reference : fl_lib/Electrical/Electrical Elements/Electrical Reference
  PS-Simulink Converter{,1..5} (6 alike) : nesl_utility/PS-Simulink Converter  PhysicalDomain=network_engine_domain  SubClassName=ps_output  LeftPortType=input  RightPortType=output  PseudoPeriodic=off  Frequencies=[]  Unit=1  AffineConversion=off
  Solver Configuration : nesl_utility/Solver Configuration  PhysicalDomain=network_engine_domain  SubClassName=solver  LeftPortType=input  RightPortType=generic  Tones=[]  Harmonics=[]  SimulateNoise=off  Profile=off  UseLocalSampling=off  EnableSwitchedLinearOptims=on  FrequencyDomain=off  UseCCode=off  RelTol=0.001  AbsTol=1e-06  MinStep=1e-09  ToWorkspace=off  RevertToSquareIcSolve=off  NumHomotopyIterations=100  PhasorMode=off  PhasorModeNumHarmonics=1  DoDC=off  ResidualTolerance=1e-09  UseLocalSolver=on  LocalSolverChoice=NE_BACKWARD_EULER_ADVANCER  LocalSolverSampleTime=1e-6  DoFixedCost=on  MaxNonlinIter=3  MaxModeIter=2  ComputeImpulses=off  ImpulseIterations=2  LinearAlgebra=Sparse  EquationFormulation=NE_TIME_EF  DelaysMemoryBudget=1024  AutomaticFiltering=on  FilteringTimeConstant=0.001  PartitionStorageMethod=AS_NEEDED  PartitionMemoryBudget=1024  PartitionMethod=FAST
  Voltage Sensor{,1..5} (6 alike) : fl_lib/Electrical/Electrical Sensors/Voltage Sensor
  Voltage Source : ee_lib/Sources/Voltage Source (Three-Phase)  vline_rms=A*sqrt(3)/sqrt(2) V  shift=0 deg  freq=f Hz  impedance_option=1  SShortCircuit=1e6 V*A  XR=15  R=0.01 Ohm  L=3.97e-4 H  G_parasitic=0 1/Ohm  harmonic_option=1  harmonic_orders=Harmonic_Orders  harmonic_ratios=Harmonic_Amplitudes  I_specify=off  I_priority=None  I=[ 0 0 0 ] A  I_nominal_specify=off  I_nominal_unit=A  I_nominal_value=1
      settings: SourceProductBaseCode=PS  InternalSimscapePortConfiguration="{\"Bottom\":[],\"Left\":[{\"id\":\"n\",\"label\":\"n\",\"type\":\"foundation.electrical.electrical\"}],\"Right\":[{\"id\":\"a\",\"label\":\"a\",\"type\":\"foundation.electrical.electrical\"},{\"id\":\"b\",\"label\":\"b\",\"type\":\"foundation.electrical.electrical\"},{\"id\":\"c\",\"label\":\"c\",\"type\":\"foundation.electrical.electrical\"}],\"Top\":[]}"
  Voltage Source1 : ee_lib/Sources/Voltage Source (Three-Phase)  vline_rms=A*sqrt(3)/sqrt(2) V  shift=-30 deg  freq=f Hz  impedance_option=1  SShortCircuit=1e6 V*A  XR=15  R=0.01 Ohm  L=3.97e-4 H  G_parasitic=0 1/Ohm  harmonic_option=1  harmonic_orders=Harmonic_Orders  harmonic_ratios=Harmonic_Amplitudes  I_specify=off  I_priority=None  I=[ 0 0 0 ] A  I_nominal_specify=off  I_nominal_unit=A  I_nominal_value=1
      settings: SourceProductBaseCode=PS  InternalSimscapePortConfiguration="{\"Bottom\":[],\"Left\":[{\"id\":\"n\",\"label\":\"n\",\"type\":\"foundation.electrical.electrical\"}],\"Right\":[{\"id\":\"a\",\"label\":\"a\",\"type\":\"foundation.electrical.electrical\"},{\"id\":\"b\",\"label\":\"b\",\"type\":\"foundation.electrical.electrical\"},{\"id\":\"c\",\"label\":\"c\",\"type\":\"foundation.electrical.electrical\"}],\"Top\":[]}"
  output : Outport
  output1 : Outport  Port=2
  output2 : Outport  Port=3
  output3 : Outport  Port=4
  output4 : Outport  Port=5
  output5 : Outport  Port=6
  wires:
  PS-Simulink Converter2/1 -> output2/1
  PS-Simulink Converter5/1 -> output5/1
  PS-Simulink Converter1/1 -> output1/1
  PS-Simulink Converter4/1 -> output4/1
  PS-Simulink Converter3/1 -> output3/1
  PS-Simulink Converter/1 -> output/1
  connections:
  Voltage Source/RConn2 -- Voltage Sensor1/LConn1
  Voltage Sensor/LConn1 -- Voltage Source/RConn1
  PS-Simulink Converter3/LConn1 -- Voltage Sensor3/RConn1
  PS-Simulink Converter2/LConn1 -- Voltage Sensor2/RConn1
  Voltage Sensor2/LConn1 -- Voltage Source/RConn3
  PS-Simulink Converter4/LConn1 -- Voltage Sensor4/RConn1
  Voltage Sensor5/LConn1 -- Voltage Source1/RConn3
  Voltage Source1/RConn2 -- Voltage Sensor4/LConn1
  PS-Simulink Converter/LConn1 -- Voltage Sensor/RConn1
  Voltage Sensor3/LConn1 -- Voltage Source1/RConn1
  PS-Simulink Converter1/LConn1 -- Voltage Sensor1/RConn1
  PS-Simulink Converter5/LConn1 -- Voltage Sensor5/RConn1
  Voltage Sensor4/RConn2 -- Voltage Sensor3/RConn2 -- Voltage Source1/LConn1 -- Electrical Reference/LConn1 -- Voltage Sensor/RConn2 -- Voltage Sensor1/RConn2 -- Voltage Sensor2/RConn2 -- Voltage Source/LConn1 -- Solver Configuration/RConn1 -- Voltage Sensor5/RConn2

== system gm_external_state_machine/Subsystem1 ==
  note: 6-phase 2-level inverter
  note: electrical motor and mechanical system
  In1 : Inport
  10kHz_current : Scope
  6ph_Inverter : Subsystem
  Constant30 : Constant  Value=2*pi  SampleTime=-1
  Constant44 : Constant  Value=v_dc  SampleTime=-1
  DC_link : Subsystem
  Data Type Conversion66 : DataTypeConversion  OutDataTypeStr=double
  Demux2 : Demux  Outputs=12
  Electrical Reference1 : fl_lib/Electrical/Electrical Elements/Electrical Reference
  Gain1 : Gain  Gain=30/pi
  Gain2 : Gain  Gain=pi/30
  Gain7 : Gain  Gain=p
  Ideal Angular Velocity Source1 : fl_lib/Mechanical/Mechanical Sources/Ideal Angular Velocity Source
  Ideal Rotational Motion Sensor1 : fl_lib/Mechanical/Mechanical Sensors/Ideal Rotational Motion Sensor  wrap_angle=simscape.enum.onoff.off  offset=0 deg
  Inertia1 : fl_lib/Mechanical/Rotational Elements/Inertia  inertia=J kg*m^2  num_ports=foundation.enum.numPorts2.one  w_specify=off  w_priority=High  w=0 rad/s  w_nominal_specify=off  w_nominal_unit=rad/s  w_nominal_value=1  t_specify=off  t_priority=None  t=0 N*m  t_nominal_specify=off  t_nominal_unit=N*m  t_nominal_value=1
  Mechanical Rotational Reference1 : fl_lib/Mechanical/Rotational Elements/Mechanical Rotational Reference
  Mod : Math  Operator=mod  SaturateOnIntegerOverflow=on
  Mux8 : Mux  Inputs=6
  Open Circuit : fl_lib/Electrical/Electrical Elements/Open Circuit  v_specify=off  v_priority=None  v=0 V  v_nominal_specify=off  v_nominal_unit=V  v_nominal_value=1
      settings: SourceProductBaseCode=SS
  Open Circuit1 : fl_lib/Electrical/Electrical Elements/Open Circuit  v_specify=off  v_priority=None  v=0 V  v_nominal_specify=off  v_nominal_unit=V  v_nominal_value=1
      settings: SourceProductBaseCode=SS
  PS-Simulink Converter6 : nesl_utility/PS-Simulink Converter  PhysicalDomain=network_engine_domain  SubClassName=ps_output  LeftPortType=input  RightPortType=output  PseudoPeriodic=off  Frequencies=[]  Unit=1  AffineConversion=off
      settings: SourceProductBaseCode=PW,SS
  PS-Simulink Converter7 : nesl_utility/PS-Simulink Converter  PhysicalDomain=network_engine_domain  SubClassName=ps_output  LeftPortType=input  RightPortType=output  PseudoPeriodic=off  Frequencies=[]  Unit=1  AffineConversion=off
      settings: SourceProductBaseCode=PW,SS
  Power_Source : Subsystem
  Rate Transition : RateTransition  OutPortSampleTime=1e-6
  Rate Transition67 : RateTransition  OutPortSampleTime=0.0001
  Simscape Component : SimscapeComponentBlock  SourceFile=SixPhase_PMSM  ComponentPath=SixPhase_PMSM  ComponentVariants=SixPhase_PMSM  ComponentVariantNames=SixPhase_PMSM  ClassName=SixPhase_PMSM  SchemaVersion=1  Rs=Rs Ohm  Ld=Ld H  Lq=Lq H  Lx=Lx H  Ly=Ly H  psiPM=psi_pm Wb  np=p  theta_m_specify=off  theta_m_priority=None  theta_m=0 rad  theta_m_nominal_specify=off  theta_m_nominal_unit=rad  theta_m_nominal_value=1
      settings: CopyFcn=simscape.engine.sli.internal.componentblockcallback(gcbh,'COPY')  PreCopyFcn=simscape.engine.sli.internal.componentblockcallback(gcbh,'PRECOPY')  PreDeleteFcn=simscape.engine.sli.internal.componentblockcallback(gcbh,'PREDELETE')  InternalSimscapePortConfiguration="{\"Bottom\":[],\"Left\":[{\"id\":\"a1\",\"label\":\"a1\",\"type\":\"foundation.electrical.electrical\"},{\"id\":\"b1\",\"label\":\"b1\",\"type\":\"foundation.electrical.electrical\"},{\"id\":\"c1\",\"label\":\"c1\",\"type\":\"foundation.electrical.electrical\"},{\"id\":\"a2\",\"label\":\"a2\",\"type\":\"foundation.electrical.electrical\"},{\"id\":\"b2\",\"label\":\"b2\",\"type\":\"foundation.electrical.electrical\"},{\"id\":\"c2\",\"label\":\"c2\",\"type\":\"foundation.electrical.electrical\"},{\"id\":\"n1\",\"label\":\"n1\",\"type\":\"foundation.electrical.electrical\"},{\"id\":\"n2\",\"label\":\"n2\",\"type\":\"foundation.electrical.electrical\"}],\"Right\":[{\"id\":\"R\",\"label\":\"R\",\"type\":\"foundation.mechanical.rotational.rotational\"},{\"id\":\"C\",\"label\":\"C\",\"type\":\"foundation.mechanical.rotational.rotational\"}],\"Top\":[]}"
      mask Type: SixPhase_PMSM
  Simulink-PS Converter{,2..8,11..12,17..20} (14 alike) : nesl_utility/Simulink-PS Converter  PhysicalDomain=network_engine_domain  SubClassName=ps_input  LeftPortType=input  RightPortType=output  PseudoPeriodic=off  Frequencies=[]  NoiseDistribution=none  NoiseParameters=[]  Unit=1  AffineConversion=off  FilteringAndDerivatives=provide  SimscapeFilterOrder=1  InputFilterTimeConstant=0.001  UdotUserProvided=0
      Simulink-PS Converter settings: SourceProductBaseCode=PW,SS
      Simulink-PS Converter8 settings: SourceProductBaseCode=PW,SS
  Solver Configuration1 : nesl_utility/Solver Configuration  PhysicalDomain=network_engine_domain  SubClassName=solver  LeftPortType=input  RightPortType=generic  Tones=[]  Harmonics=[]  SimulateNoise=off  Profile=off  UseLocalSampling=off  EnableSwitchedLinearOptims=on  FrequencyDomain=off  UseCCode=off  RelTol=0.001  AbsTol=1e-06  MinStep=1e-09  ToWorkspace=off  RevertToSquareIcSolve=off  NumHomotopyIterations=100  PhasorMode=off  PhasorModeNumHarmonics=1  DoDC=off  ResidualTolerance=1e-09  UseLocalSolver=on  LocalSolverChoice=NE_BACKWARD_EULER_ADVANCER  LocalSolverSampleTime=1e-6  DoFixedCost=on  MaxNonlinIter=3  MaxModeIter=2  ComputeImpulses=off  ImpulseIterations=2  LinearAlgebra=Sparse  EquationFormulation=NE_TIME_EF  DelaysMemoryBudget=1024  AutomaticFiltering=on  FilteringTimeConstant=0.001  PartitionStorageMethod=AS_NEEDED  PartitionMemoryBudget=1024  PartitionMethod=FAST
      settings: SourceProductBaseCode=PW,SS
  n_ref : Constant  Value=n_rpm  SampleTime=-1
  i_ph : Outport
  i_dc : Outport  Port=2
  theta_el : Outport  Port=3
  omega_m : Outport  Port=4
  wires:
  6ph_Inverter/7(u_1_gnd) -> ?  "i_dc"
  Rate Transition67/1 -> 10kHz_current/1
  Demux2/3 -> Simulink-PS Converter5/1
  n_ref/1 -> Gain2/1
  6ph_Inverter/6(i_6) -> Mux8/6  "i_c2"
  Rate Transition/1 -> Data Type Conversion66/1
  Demux2/8 -> Simulink-PS Converter19/1
  6ph_Inverter/4(i_4) -> Mux8/4  "i_a2"
  Demux2/10 -> Simulink-PS Converter3/1
  Demux2/2 -> Simulink-PS Converter4/1
  Demux2/1 -> Simulink-PS Converter2/1
  Constant44/1 -> Simulink-PS Converter/1
  6ph_Inverter/1(i_1) -> Mux8/1  "i_a1"
  Demux2/7 -> Simulink-PS Converter18/1
  Constant30/1 -> Mod/2
  Demux2/9 -> Simulink-PS Converter20/1
  Demux2/4 -> Simulink-PS Converter6/1
  Demux2/12 -> Simulink-PS Converter12/1
  In1/1 -> Rate Transition/1
  DC_link/1(u_dc_link_measured) -> [u_dc_link]
  6ph_Inverter/2(i_2) -> Mux8/2  "i_b1"
  Mod/1 -> [theta_el], theta_el/1
  Data Type Conversion66/1 -> Demux2/1
  PS-Simulink Converter7/1 -> Gain7/1  "theta_m"
  6ph_Inverter/13(i_dc) -> [i_dc], i_dc/1
  Demux2/5 -> Simulink-PS Converter7/1
  Demux2/6 -> Simulink-PS Converter17/1
  Gain1/1 -> [n_RPM]
  PS-Simulink Converter6/1 -> Gain1/1  "omega_m"
  6ph_Inverter/5(i_5) -> Mux8/5  "i_b2"
  6ph_Inverter/3(i_3) -> Mux8/3  "i_c1"
  Gain7/1 -> Mod/1  "theta_el"
  Gain2/1 -> Simulink-PS Converter8/1, omega_m/1, [omega_m]
  Demux2/11 -> Simulink-PS Converter11/1
  Mux8/1 -> [i_ph], i_ph/1, Rate Transition67/1
  connections:
  Simulink-PS Converter20/RConn1 -- 6ph_Inverter/LConn9
  Simulink-PS Converter2/RConn1 -- 6ph_Inverter/LConn1
  Simulink-PS Converter18/RConn1 -- 6ph_Inverter/LConn7
  6ph_Inverter/RConn1 -- Simscape Component/LConn1
  6ph_Inverter/LConn13 -- DC_link/RConn1
  Power_Source/RConn1 -- DC_link/LConn1
  Simulink-PS Converter8/RConn1 -- Ideal Angular Velocity Source1/RConn1
  Simulink-PS Converter4/RConn1 -- 6ph_Inverter/LConn2
  6ph_Inverter/RConn5 -- Simscape Component/LConn5
  Simulink-PS Converter5/RConn1 -- 6ph_Inverter/LConn3
  PS-Simulink Converter7/LConn1 -- Ideal Rotational Motion Sensor1/RConn3
  Simulink-PS Converter19/RConn1 -- 6ph_Inverter/LConn8
  Simulink-PS Converter/RConn1 -- Power_Source/LConn1
  6ph_Inverter/RConn2 -- Simscape Component/LConn2
  Simscape Component/LConn8 -- Open Circuit1/LConn1
  Simulink-PS Converter7/RConn1 -- 6ph_Inverter/LConn5
  Simscape Component/LConn7 -- Open Circuit/LConn1
  Simulink-PS Converter17/RConn1 -- 6ph_Inverter/LConn6
  6ph_Inverter/RConn4 -- Simscape Component/LConn4
  Simulink-PS Converter12/RConn1 -- 6ph_Inverter/LConn12
  6ph_Inverter/LConn14 -- DC_link/RConn2
  Simscape Component/LConn3 -- 6ph_Inverter/RConn3
  Simulink-PS Converter11/RConn1 -- 6ph_Inverter/LConn11
  Simulink-PS Converter3/RConn1 -- 6ph_Inverter/LConn10
  Simscape Component/RConn2 -- Ideal Angular Velocity Source1/RConn2 -- Ideal Rotational Motion Sensor1/RConn1 -- Mechanical Rotational Reference1/LConn1
  Inertia1/LConn1 -- Ideal Angular Velocity Source1/LConn1 -- Simscape Component/RConn1 -- Ideal Rotational Motion Sensor1/LConn1
  Simscape Component/LConn6 -- 6ph_Inverter/RConn6
  Solver Configuration1/RConn1 -- Power_Source/RConn2 -- DC_link/LConn2 -- Electrical Reference1/LConn1
  PS-Simulink Converter6/LConn1 -- Ideal Rotational Motion Sensor1/RConn2
  Simulink-PS Converter6/RConn1 -- 6ph_Inverter/LConn4

== system gm_external_state_machine/Subsystem2 ==
  note: Since i count now every On and Off Transition for each switch,
      |  i have to divide by 12*2 in order to get the switching frequency
      |  (after dividing by the time).
      | 12 comes from the 12 switches
      | 2 comes from that 1 ON-transition and 1 OFF-transition = 1 switching-cycle
  note: 1 for one cycle if edge recognized
  note: Over AXI, 32 Bit are received.
      | However, only one Bit is used.
  note: To avoid unneccessary calcualtions, i divide by 24 on the ARM processor.
  ss_in_0 : Inport
  ss_in_1 : Inport  Port=2
  ss_in_2 : Inport  Port=3
  ss_in_3 : Inport  Port=4
  ss_in_4 : Inport  Port=5
  ss_in_5 : Inport  Port=6
  ss_in_6 : Inport  Port=7
  ss_in_7 : Inport  Port=8
  ss_in_8 : Inport  Port=9
  ss_in_9 : Inport  Port=10
  ss_in_10 : Inport  Port=11
  ss_in_11 : Inport  Port=12
  bResetAXI : Inport  Port=13
  Count_f_sw : MATLAB Function  TreatAsAtomicUnit=on  VariantControl=(default)
  Detec_edge : Sum  Inputs=+-  AccumDataTypeStr=int8  OutDataTypeStr=int8
  Gain : Gain  Commented=on  Gain=1/(12*2)
  Mux : Mux  Inputs=6
  Mux1 : Mux  Inputs=6
  Mux2 : Mux  Inputs=2
  SS_Old : Delay  DelayLength=1
  Saturation : Saturate  UpperLimit=1  LowerLimit=0  OutMin=[0]  OutMax=[1]  OutDataTypeStr=fixdt(0,1)
  Scope : Scope  NumInputPorts=2
  delay : Delay  DelayLength=1
  reset_old2 : Delay  DelayLength=1
  reset_old_switch1 : Switch  Criteria=u2 ~= 0
  switchNumb_AXI : Outport  VectorParamsAs1DForOutWhenUnconnected=off
  switchNumb : Outport  Port=2  VectorParamsAs1DForOutWhenUnconnected=off
  wires:
  Count_f_sw/1(switchNumbOut) -> switchNumb/1, switchNumb_AXI/1, delay/1
  SS_Old/1 -> Count_f_sw/2(ss_v_old)
  ss_in_3/1 -> Mux/4
  bResetAXI/1 -> Detec_edge/1, reset_old_switch1/1, Scope/2
  ss_in_7/1 -> Mux1/2
  reset_old_switch1/1 -> reset_old2/1
  Mux1/1 -> Mux2/2
  Detec_edge/1 -> reset_old_switch1/2, Saturation/1  "1 for one cycle if edge recognized"
  reset_old2/1 -> reset_old_switch1/3, Detec_edge/2
  delay/1 -> Count_f_sw/1(switchNumb)
  Mux2/1 -> Count_f_sw/3(ss_v), SS_Old/1
  ss_in_0/1 -> Mux/1
  ss_in_2/1 -> Mux/3
  Mux/1 -> Mux2/1
  ss_in_4/1 -> Mux/5
  Saturation/1 -> Scope/1, Count_f_sw/4(bReset)
  ss_in_5/1 -> Mux/6
  ss_in_1/1 -> Mux/2
  ss_in_8/1 -> Mux1/3
  ss_in_11/1 -> Mux1/6
  ss_in_10/1 -> Mux1/5
  ss_in_6/1 -> Mux1/1
  ss_in_9/1 -> Mux1/4
